simulink model "counter"  (R2018a)
settings: Solver=VariableStepAuto  StartTime=0.0  StopTime=10.0  RelTol=1e-3
settings Model: Creator=Edoardo  LastModifiedBy=Edoardo

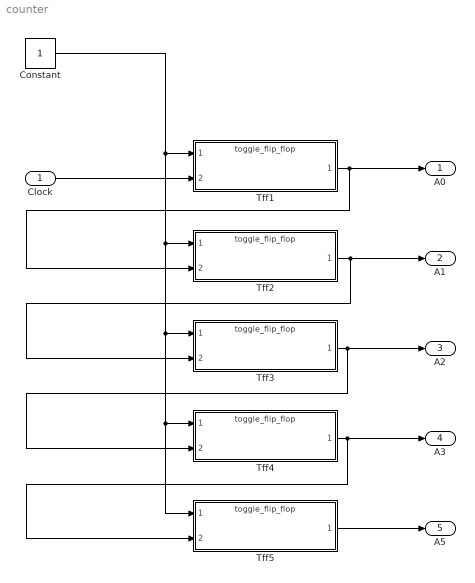
== system counter ==
  Clock : Inport
  Constant : Constant  OutDataTypeStr=boolean
  Tff{1..5} (5 alike) : ModelReference  ModelNameDialog=toggle_flip_flop.slx  SimulationMode=Normal  ModelReferenceVersion=1.10
  "A0 " : Outport
  A1 : Outport  Port=2
  A2 : Outport  Port=3
  A3 : Outport  Port=4
  A5 : Outport  Port=5
  wires:
  Constant/1 -> Tff5/1, Tff4/1, Tff3/1, Tff2/1, Tff1/1
  Tff5/1 -> A5/1
  Clock/1 -> Tff1/2
  Tff1/1 -> Tff2/2, "A0 "/1
  Tff2/1 -> Tff3/2, A1/1
  Tff3/1 -> Tff4/2, A2/1
  Tff4/1 -> Tff5/2, A3/1
